simulink model "grid"  (R2015b)
settings: Solver=FixedStepAuto  StartTime=0.0  StopTime=75  FixedStep=Ts  RelTol=1e-3
undefined symbols (not defined in the file): Ts
libraries: powerlib x10, sps_avr x2, powerlib_meascontrol x1
settings Model: Creator=Eren  LastModifiedBy=Eren

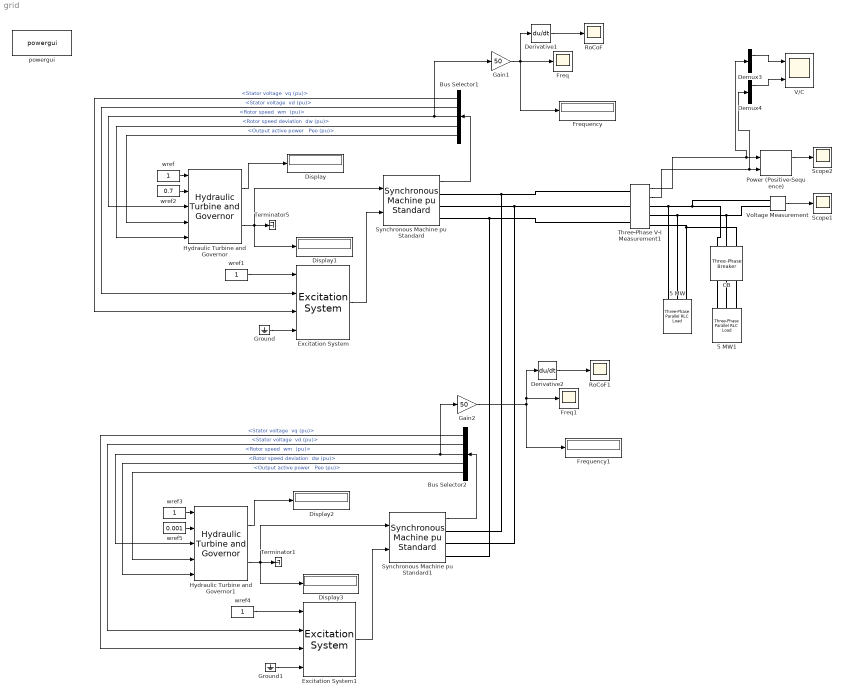
== system grid ==
  5 MW : powerlib/Elements/Three-Phase Parallel RLC Load  LConnTagsString=A|B|C  Configuration=Y (grounded)  NominalVoltage=690  Vabc=[1e3 1e3 1e3]  Vabcp=[1e3 1e3 1e3]  NominalFrequency=50  UnbalancedPower=off  ActivePower=80e6  InductivePower=0  CapacitivePower=0  Pabc=[10e3 9e3 11e3]  QLabc=[100 90 110]  QCabc=[100 90 110]  Pabcp=[10e3 9e3 11e3]  QLabcp=[100 90 110]  QCabcp=[100 90 110]  Measurements=None  LoadType=constant PQ
  5 MW1 : powerlib/Elements/Three-Phase Parallel RLC Load  LConnTagsString=A|B|C  Configuration=Y (grounded)  NominalVoltage=690  Vabc=[1e3 1e3 1e3]  Vabcp=[1e3 1e3 1e3]  NominalFrequency=50  UnbalancedPower=off  ActivePower=16e6  InductivePower=0  CapacitivePower=0  Pabc=[10e3 9e3 11e3]  QLabc=[100 90 110]  QCabc=[100 90 110]  Pabcp=[10e3 9e3 11e3]  QLabcp=[100 90 110]  QCabcp=[100 90 110]  Measurements=None  LoadType=constant PQ
  Bus Selector1 : BusSelector  OutputSignals="dq0 components.Stator voltage  vq (pu),dq0 components.Stator voltage  vd (pu),Mechanical.Rotor speed  wm  (pu),Mechanical.Rotor speed deviation  dw (pu),Output active power   Peo (pu)"
  Bus Selector2 : BusSelector  OutputSignals="dq0 components.Stator voltage  vq (pu),dq0 components.Stator voltage  vd (pu),Mechanical.Rotor speed  wm  (pu),Mechanical.Rotor speed deviation  dw (pu),Output active power   Peo (pu)"
  CB : powerlib/Elements/Three-Phase Breaker  InitialState=open  SwitchA=on  SwitchB=on  SwitchC=on  SwitchTimes="[34  76]"  External=off  BreakerResistance=0.01  SnubberResistance=1e6  SnubberCapacitance=inf  Measurements=None
  Demux3 : Demux  Outputs=3
  Demux4 : Demux  Outputs=3
  Derivative1 : Derivative
  Derivative2 : Derivative
  Display{,1..3} (4 alike) : Display
  Excitation System : sps_avr/Excitation System  tr=20e-3  reg=[ 350, 0.001 ]  exc=[ 1, 0 ]  tgr=[ 0, 0 ]  damp=[ 0.001, 0.1 ]  sat=[ 0, 0 ]  lim=[ -11.5, 11.5, 0 ]  v0="[1.0  1.28]"
  Excitation System1 : sps_avr/Excitation System  tr=20e-3  reg=[ 350, 0.001 ]  exc=[ 1, 0 ]  tgr=[ 0, 0 ]  damp=[ 0.001, 0.1 ]  sat=[ 0, 0 ]  lim=[ -11.5, 11.5, 0 ]  v0="[1.0  1.28]"
  Freq : Scope
  Freq1 : Scope
  Frequency : Display
  Frequency1 : Display
  Gain1 : Gain  Gain=50
  Gain2 : Gain  Gain=50
  Ground : Ground
  Ground1 : Ground
  Hydraulic Turbine and Governor : powerlib/Machines/Hydraulic Turbine and Governor  sm="[ 10/3  0.07 ]"  gate="[  0.01  1.2  -0.2  0.2 ]"  reg="[  0.04  10  0.105  0  0.01  ]"  hyd="[  0  2.67  ]"  dref=0  po=0.7
  Hydraulic Turbine and Governor1 : powerlib/Machines/Hydraulic Turbine and Governor  sm="[ 10/3  0.07 ]"  gate="[  0.001  1.2  -0.2  0.2 ]"  reg="[  0.04  10  0.105  0  0.01  ]"  hyd="[  0  2.67  ]"  dref=0  po=0.001
  Power (Positive-Sequence) : powerlib_meascontrol/Measurements/Power (Positive-Sequence)  Freq=60  Vinit=[0, 0]  Iinit=[0, 0]  Ts=0
  RoCoF : Scope
  RoCoF1 : Scope
  Scope1 : Scope
  Scope2 : Scope
  Synchronous Machine pu Standard : powerlib/Machines/Synchronous Machine pu Standard  PresetModel=No  MechanicalLoad=Mechanical power Pm  ShowDetailedParameters=on  RotorType=Round  Units=per unit standard parameters  MeasurementBus=off  NominalParameters=[100e+06 690 50]  Reactances1=[ 1.81, 0.3, 0.23, 1.76, 0.65, 0.25, 0.15 ]  Reactances2=[2.24 0.17 0.12 1.02 0.13 0.08]  dAxisTimeConstants=Short-circuit  qAxisTimeConstants=Short-circuit  TimeConstants1="[ 4.4849  0.0681  0.1  ]"  TimeConstants2=[ 8.0, 0.03, 1.0, 0.07 ]  TimeConstants3="[  4.49  0.0681  0.0513  ]"  TimeConstants4=[ 8.0, 0.03, 0.3371, 0.0295 ]  TimeConstants5=[ 1.01, 0.053, 0.1 ]  TimeConstants6=[ 1.3201, 0.023, 1.0, 0.07 ]  TimeConstants7=[0.012 0.003 0.003]  TimeConstants8=[ 1.3201, 0.0231, 0.3371, 0.0295 ]  StatorResistance=0.000037875  Mechanical=[5 0.02056 4]  PolePairs=20  InitialConditions="[ 0  0  0  0  0  0  0  0  1 ]"  SetSaturation=off  Saturation=[0.6404,0.7127,0.8441,0.9214,0.9956,1.082,1.19,1.316,1.457;0.7,0.7698,0.8872,0.9466,0.9969,1.046,1.1,1.151,1.201]  LoadFlowParameters=[1,0,0,0,0]  TsPowergui=0  TsBlock=-1  IterativeModel=Trapezoidal non iterative  BusType=swing  Pref=0  Qref=0  Qmin=-inf  Qmax=inf  PLF=0  QLF=0
  Synchronous Machine pu Standard1 : powerlib/Machines/Synchronous Machine pu Standard  PresetModel=No  MechanicalLoad=Mechanical power Pm  ShowDetailedParameters=on  RotorType=Round  Units=per unit standard parameters  MeasurementBus=off  NominalParameters=[100e+06 690 50]  Reactances1=[ 1.81, 0.3, 0.23, 1.76, 0.65, 0.25, 0.15 ]  Reactances2=[2.24 0.17 0.12 1.02 0.13 0.08]  dAxisTimeConstants=Short-circuit  qAxisTimeConstants=Short-circuit  TimeConstants1="[ 4.4849  0.0681  0.1  ]"  TimeConstants2=[ 8.0, 0.03, 1.0, 0.07 ]  TimeConstants3="[  4.49  0.0681  0.0513  ]"  TimeConstants4=[ 8.0, 0.03, 0.3371, 0.0295 ]  TimeConstants5=[ 1.01, 0.053, 0.1 ]  TimeConstants6=[ 1.3201, 0.023, 1.0, 0.07 ]  TimeConstants7=[0.012 0.003 0.003]  TimeConstants8=[ 1.3201, 0.0231, 0.3371, 0.0295 ]  StatorResistance=0.000037875  Mechanical=[5 0.02056 4]  PolePairs=20  InitialConditions="[ 0  0  0  0  0  0  0  0  1 ]"  SetSaturation=off  Saturation=[0.6404,0.7127,0.8441,0.9214,0.9956,1.082,1.19,1.316,1.457;0.7,0.7698,0.8872,0.9466,0.9969,1.046,1.1,1.151,1.201]  LoadFlowParameters=[1,0,0,0,0]  TsPowergui=0  TsBlock=-1  IterativeModel=Trapezoidal non iterative  BusType=swing  Pref=0  Qref=0  Qmin=-inf  Qmax=inf  PLF=0  QLF=0
  Terminator1 : Terminator
  Terminator5 : Terminator
  Three-Phase V-I Measurement1 : powerlib/Measurements/Three-Phase V-I Measurement  VoltageMeasurement=phase-to-ground  SetLabelV=off  LabelV=Vsabc  Vpu=off  VpuLL=on  CurrentMeasurement=yes  SetLabelI=off  LabelI=Isabc  Ipu=off  Pbase=100e6  Vbase=690  OutputType=Complex  PhasorSimulation=off  PSBequivalent=0
  "V/C " : Scope  NumInputPorts=2
  Voltage Measurement : powerlib/Measurements/Voltage Measurement  PhasorSimulation=off  OutputType=Complex  PSBequivalent=0
  powergui : powerlib/powergui  Priority=2  SimulationMode=Discrete  SolverType=Tustin  SampleTime=Ts  frequency=60  SPID=off  DisableSnubberDevices=off  DisableRonSwitches=off  DisableVfSwitches=off  SwTol=0  DisplayEquations=off  Interpol=off  ExternalGateDelay=off  methode=off  Ts=0  FunctionMessages=off  echomessages=off  HookPort=off  EnableUseOfTLC=off  x0status=blocks  frequencyindice=50  Pbase=100e6  ErrMax=1e-4  Iterations=50  UnitsV=kV  UnitsW=MW  buscounter=0  RestoreLinks=warning  ResistiveCurrentMeasurement=off  Frange=[0:2:500]  Ylog=off  Xlog=on  ShowGrid=off  save=off  variable=ZData  structure=0  ZoomFFT=on  StartTime=0.0  cycles=1  DisplayStyle=1  fundamental=60  FreqAxis=off  MaxFrequency=1000  frequencyindicesteady=1  RmsSteady=1  display=off
  wref{,1,3..4} (4 alike) : Constant
  wref2 : Constant  Value=0.7
  wref5 : Constant  Value=0.001
  wires:
  Synchronous Machine pu Standard/1 -> Bus Selector1/1
  Bus Selector1/3 -> Gain1/1, Hydraulic Turbine and Governor/3  "<Rotor speed  wm  (pu)>"
  Bus Selector1/4 -> Hydraulic Turbine and Governor/5  "<Rotor speed deviation  dw (pu)>"
  Bus Selector1/5 -> Hydraulic Turbine and Governor/4  "<Output active power   Peo (pu)>"
  Excitation System/1 -> Synchronous Machine pu Standard/2
  Bus Selector1/2 -> Excitation System/2  "<Stator voltage  vd (pu)>"
  Bus Selector1/1 -> Excitation System/3  "<Stator voltage  vq (pu)>"
  Hydraulic Turbine and Governor/2 -> Synchronous Machine pu Standard/1, Display1/1, Terminator5/1
  wref/1 -> Hydraulic Turbine and Governor/1
  Ground/1 -> Excitation System/4
  wref1/1 -> Excitation System/1
  wref2/1 -> Hydraulic Turbine and Governor/2
  Voltage Measurement/1 -> Scope1/1
  Three-Phase V-I Measurement1/1 -> Demux3/1, Power (Positive-Sequence)/1
  Three-Phase V-I Measurement1/2 -> Demux4/1, Power (Positive-Sequence)/2
  Power (Positive-Sequence)/1 -> Scope2/1
  Hydraulic Turbine and Governor/1 -> Display/1
  Gain1/1 -> Derivative1/1, Frequency/1, Freq/1
  Derivative1/1 -> RoCoF/1
  Demux4/1 -> "V/C "/2
  Demux3/1 -> "V/C "/1
  Synchronous Machine pu Standard1/1 -> Bus Selector2/1
  Bus Selector2/3 -> Gain2/1, Hydraulic Turbine and Governor1/3  "<Rotor speed  wm  (pu)>"
  Bus Selector2/4 -> Hydraulic Turbine and Governor1/5  "<Rotor speed deviation  dw (pu)>"
  Bus Selector2/5 -> Hydraulic Turbine and Governor1/4  "<Output active power   Peo (pu)>"
  Excitation System1/1 -> Synchronous Machine pu Standard1/2
  Bus Selector2/2 -> Excitation System1/2  "<Stator voltage  vd (pu)>"
  Bus Selector2/1 -> Excitation System1/3  "<Stator voltage  vq (pu)>"
  Hydraulic Turbine and Governor1/2 -> Synchronous Machine pu Standard1/1, Display3/1, Terminator1/1
  wref3/1 -> Hydraulic Turbine and Governor1/1
  Ground1/1 -> Excitation System1/4
  wref4/1 -> Excitation System1/1
  wref5/1 -> Hydraulic Turbine and Governor1/2
  Hydraulic Turbine and Governor1/1 -> Display2/1
  Gain2/1 -> Derivative2/1, Freq1/1, Frequency1/1
  Derivative2/1 -> RoCoF1/1
  connections:
  5 MW/LConn1 -- Three-Phase V-I Measurement1/RConn1 -- CB/RConn1 -- Voltage Measurement/LConn1
  5 MW/LConn2 -- Three-Phase V-I Measurement1/RConn2 -- CB/RConn2 -- Voltage Measurement/LConn2
  Three-Phase V-I Measurement1/RConn3 -- CB/RConn3 -- 5 MW/LConn3
  Three-Phase V-I Measurement1/LConn3 -- Synchronous Machine pu Standard1/RConn3 -- Synchronous Machine pu Standard/RConn3
  Synchronous Machine pu Standard/RConn2 -- Three-Phase V-I Measurement1/LConn2 -- Synchronous Machine pu Standard1/RConn2
  Three-Phase V-I Measurement1/LConn1 -- Synchronous Machine pu Standard1/RConn1 -- Synchronous Machine pu Standard/RConn1
  CB/LConn2 -- 5 MW1/LConn2
  CB/LConn1 -- 5 MW1/LConn1
  CB/LConn3 -- 5 MW1/LConn3
